simulink model "MSM_strain_wave_actuator"  (R2024b)
settings: Solver=ode23t  StartTime=0.0  StopTime=SIMULATION_TIME  FixedStep=MAX_TIME_STEP  MaxStep=MAX_TIME_STEP  RelTol=1e-3  AbsTol=1e-3  EnableMultiTasking=on
PreLoadFcn:
  | linear_mechanism = Simulink.Variant('motion_type == "linear"');
  | rotary_mechanism = Simulink.Variant('motion_type == "rotary"');
values from neighbouring files (symbols this model uses):
  action = round(out.position_data.Data(:,5))    [msm_tooth_training_run.m]
  contact_ratio = tooth_plates_cnt / (2 * (t_a / t_b + 1))    (= 2)    [MSM_mechanism_simulation_properties.m]
  contraction_initial = -msm_length * e_initial    (= -0.001)    [MSM_mechanism_simulation_properties.m]
  controller_type_vec = zeros(tooth_plates_cnt, 1)    [MSM_mechanism_simulation_properties.m]
  controller_velocity_setpoint = velocity_iter    [controller_mass_comparison_runs.m]
  disk_diameter = disk_teeth_count * tooth_pitch / pi    [MSM_mechanism_simulation_properties.m]    (also in msm_sim_runs_for_pid.m = evalin('base','disk_diameter'); save_sim_result.m = evalin('base','disk_diameter'))
  disk_height = 2.5e-4    (= 0.00025)    [MSM_mechanism_simulation_properties.m]    (also in get_tooth_properties.m)
  feedback_threshold = 1.025    [MSM_mechanism_simulation_properties.m]    (also in get_tooth_properties.m; msm_sim_runs_for_pid.m = evalin('base','feedback_threshold'))
  force_control_coeff = 1.0    (= 1)    [MSM_mechanism_simulation_properties.m]
  HALT_VELOCITY = 0.2    [MSM_mechanism_simulation_properties.m]    (also in get_tooth_properties.m)
  in_pair_angle_tooth_plates_pitch = 2*pi * (-2*tooth_pitch + in_pair_tooth_plates_pitch) / (pi*disk_diameter)    (= 0.412285714286)    [MSM_mechanism_simulation_properties.m]    (also in get_tooth_properties.m = 2*pi * (-2*tooth_pitch + in_pair_tooth_plates_pitch) / (pi*t)
  MAX_OVERLOAD_VELOCITY = 100    [MSM_mechanism_simulation_properties.m]    (also in get_tooth_properties.m)
  MAX_POSITION = rack_initial_position + max_teeth_passed * tooth_plates_cnt * angle_single_tooth_step    [MSM_mechanism_simulation_properties.m]    (also in get_tooth_properties.m)
  MAX_TIME_STEP = 5e-6    (= 5e-06)    [MSM_mechanism_simulation_properties.m]
  min_tooth_motion_range = -msm_length * allowed_elongation    (= -0.001)    [MSM_mechanism_simulation_properties.m]
  motion_type_number = NaN    [MSM_mechanism_simulation_properties.m]
  next_vec_fraction = -0.05    [MSM_mechanism_simulation_properties.m]    (also in msm_sim_runs_for_pid.m = evalin('base','next_vec_fraction'))
  obs_matrix = zeros(tooth_plates_cnt, obs_matrix_size)    [MSM_mechanism_simulation_properties.m]
  one_side_absolute_offset = one_side_elongation_capacity * msm_length    (= 0.0001)    [MSM_mechanism_simulation_properties.m]
  rack_coulumb_friction = 0.05    [MSM_mechanism_simulation_properties.m]
  rack_initial_position = rack_initial_position + 4*angle_single_tooth_step    (= 0.0554357142857)    [MSM_mechanism_simulation_properties.m]    (also in get_tooth_properties.m = rack_initial_position + 4*angle_single_tooth_step)
  rack_mass = 4e-3    (= 0.004)    [MSM_mechanism_simulation_properties.m]
  rotational_rack_coulumb_friction = rack_coulumb_friction * disk_diameter    (= 0.00175)    [MSM_mechanism_simulation_properties.m]
  SIMULATION_TIME = 0.06    [MSM_mechanism_simulation_properties.m]    (also in msm_actuation_time_sensetivity.m = 0.04; msm_sim_runs_for_pid.m = evalin('base','SIMULATION_TIME'); msm_simulation_run.m = 0.08; msm_tooth_training_run.m = 0.04)
  swing_block_tooth_plates_pitch = 2 * tooth_pitch * 22 + tooth_pitch / tooth_plates_cnt    (= 0.0172575)    [MSM_mechanism_simulation_properties.m]    (also in get_tooth_properties.m = 2 * tooth_pitch * 22 + tooth_pitch / tooth_plates_cnt)
  tooth_disk_mass = 5e-3    (= 0.005)    [MSM_mechanism_simulation_properties.m]
  tooth_pitch = tooth_pitch * tooth_size_modifier    (= 0.00039)    [MSM_mechanism_simulation_properties.m]    (also in get_tooth_properties.m = 0.00024661; msm_sim_runs_for_pid.m = evalin('base','tooth_pitch'); save_sim_result.m = evalin('base','tooth_pitch'))
  tooth_plates_cnt = 4    [MSM_mechanism_simulation_properties.m]    (also in MSM_simulation_data_processing.m = sim_data.tooth_plates_cnt; msm_actuation_time_sensetivity.m = plates_cnt_iter; msm_sim_runs_for_pid.m = evalin('base','tooth_plates_cnt'); msm_simulation_run.m = plates_cnt_iter)
  tooth_plates_pitch = tooth_pitch * 12 + tooth_pitch / tooth_plates_cnt    (= 0.0047775)    [MSM_mechanism_simulation_properties.m]    (also in get_tooth_properties.m = tooth_pitch * 12 + tooth_pitch / tooth_plates_cnt)
  useful_load = -2    [MSM_mechanism_simulation_properties.m]    (also in controller_mass_comparison_runs.m)
  useful_mass = 0.0001    [MSM_mechanism_simulation_properties.m]    (also in controller_mass_comparison_runs.m = 0.025)
  VALIDATION_START_TIME = 0.25*SIMULATION_TIME    (= 0.015)    [MSM_mechanism_simulation_properties.m]
  Z = griddata(x,y,z,X,Y)    [MSM_simulation_data_processing.m]
undefined symbols (not defined in the file or in its folder): controller_amplitude_setpoint, controller_desired_profile_type, controller_frequency_setpoint, controller_loop_type, enable_neighbours_obs, enable_vel_setpoint, external_control_value, has_external_controller, initial_spike_force, random_delay_probablity, random_switch_probability, sim_state_code, simulation_pause_time, X, Y
libraries: sm_lib x141, MSM_element x72, Flat_tooth_plate x36, Rotary_tooth_plate x36, Swing_mechanism x18, nesl_utility x16, simulink x10, fl_lib x9, rllib x7, spsMeanLib x2, slctrl_autotuning x2, slpidlib x1
(part 3 of 7)

== system MSM_strain_wave_actuator/controller/Closed//open loop simple feedback controller1 ==
  rack position : Inport
  position mapping : Inport  Port=2
  initial spike : Inport  Port=3
  VEC: Feedback threshold and next vec fraction : Inport  Port=4
  Velocity setpoint : Inport  Port=5
  Clock : Clock
  Constant : Constant  Value=tooth_pitch
  Constant1 : Constant  Value=1.5*MAX_TIME_STEP
  Data Type Conversion : DataTypeConversion  OutDataTypeStr=double  RndMeth=Round  SaturateOnIntegerOverflow=off
  Delay1 : Delay  DelayLength=1  InitialCondition=1
  Demux : Demux  Outputs=2
  Gain1 : Gain  Gain=force_control_coeff
  Loop type control : Constant  Value=controller_loop_type
  MATLAB Function : MATLAB Function  TreatAsAtomicUnit=on
  Relational Operator : RelationalOperator  Operator=~=  OutDataTypeStr=boolean  RndMeth=Simplest  InputSameDT=off
  Velocity to frequency : Product  Inputs=*/
  Control Input : Outport
  signal switch spike : Outport  Port=2
  wires:
  Constant1/1 -> MATLAB Function/4(initial_idle_time)
  Velocity to frequency/1 -> MATLAB Function/3(cycle_length)
  Loop type control/1 -> MATLAB Function/2(loop_type)
  MATLAB Function/1(output_vector) -> Gain1/1
  rack position/1 -> MATLAB Function/8(rack_position)
  MATLAB Function/2(cur_active_output) -> Delay1/1, Relational Operator/1
  Delay1/1 -> Relational Operator/2, MATLAB Function/10(currently_active)
  Clock/1 -> MATLAB Function/1(time)
  initial spike/1 -> MATLAB Function/9(ticks_cnt)
  position mapping/1 -> MATLAB Function/7(feedback)
  Gain1/1 -> Control Input/1
  Constant/1 -> Velocity to frequency/1
  Velocity setpoint/1 -> Velocity to frequency/2
  Demux/1 -> MATLAB Function/5(feedback_threshold)
  Demux/2 -> MATLAB Function/6(next_vec_fraction)
  VEC: Feedback threshold and next vec fraction/1 -> Demux/1
  Relational Operator/1 -> Data Type Conversion/1
  Data Type Conversion/1 -> signal switch spike/1

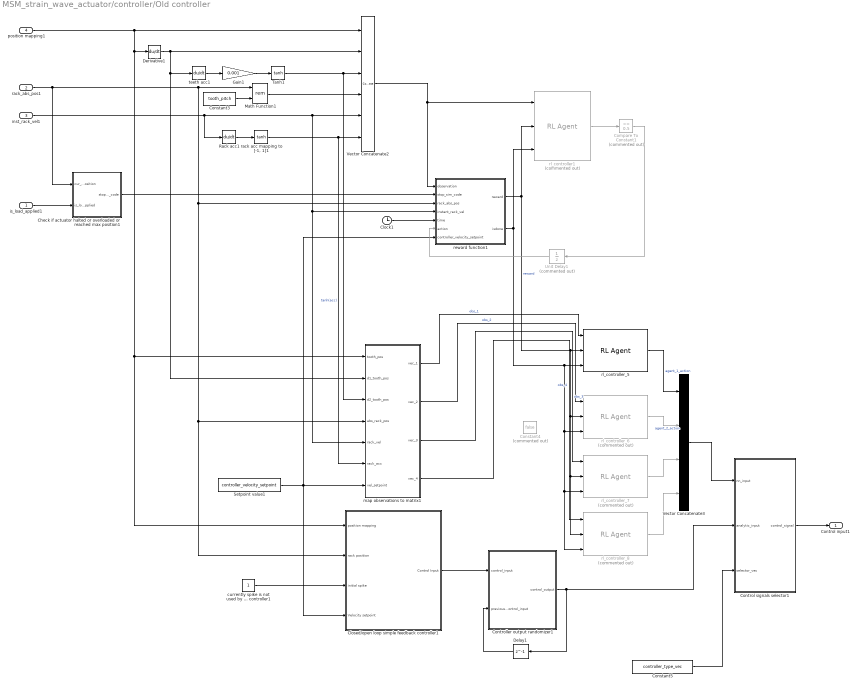
== system MSM_strain_wave_actuator/controller/Old controller ==
  is_load_applied1 : Inport
  rack_abs_pos1 : Inport  Port=2
  inst_rack_vel1 : Inport  Port=3
  position mapping1 : Inport  Port=4
  Check if actuator halted or overloaded or reached max position1 : Subsystem
  Clock1 : Clock
  Closed/open loop simple feedback controller1 : Subsystem
  Compare To Constant1 : simulink/Logic and Bit Operations/Compare To Constant  Commented=on  relop=>=  const=0.5  OutDataTypeStr=uint8
  Constant3 : Constant  Value=tooth_pitch
  Constant4 : Constant  Commented=on  Value=false
  Constant5 : Constant  Value=controller_type_vec
  Control signals selector1 : MATLAB Function  TreatAsAtomicUnit=on
  Controller output randomizer1 : MATLAB Function  TreatAsAtomicUnit=on
  Delay1 : Delay  DelayLength=1  InitialCondition=zeros(tooth_plates_cnt, 1)
  Derivative1 : Derivative
  Gain1 : Gain  Gain=0.001
  Math Function1 : Math  Operator=rem
  Rack acc1 : Derivative
  Setpoint value1 : Constant  Value=controller_velocity_setpoint
  Tanh1 : Trigonometry  Operator=tanh
  Unit Delay1 : UnitDelay  Commented=on  SampleTime=-1  HasFrameUpgradeWarning=on
  Vector Concatenate2 : Concatenate  NumInputs=6
  Vector Concatenate3 : Concatenate  NumInputs=4
  currently spike is not used by the controller1 : Constant
  map observations to matrix1 : MATLAB Function  TreatAsAtomicUnit=on
  "rack acc mapping to [-1, 1]1" : Trigonometry  Operator=tanh
  reward function1 : MATLAB Function  TreatAsAtomicUnit=on
  rl_controller1 : rllib/RL Agent  Commented=on  Agent=agent  ExternalActionAsInput=off  ProvideLastAction=off  ProvideCumRwd=off  TreatAsDirectFeedthrough=on  UseStrictObservationDataTypes=off
  rl_controller_5 : rllib/RL Agent  Agent=agent  ExternalActionAsInput=off  ProvideLastAction=off  ProvideCumRwd=off  TreatAsDirectFeedthrough=on  UseStrictObservationDataTypes=off
  rl_controller_6 : rllib/RL Agent  Commented=on  Agent=agent  ExternalActionAsInput=off  ProvideLastAction=off  ProvideCumRwd=off  TreatAsDirectFeedthrough=on  UseStrictObservationDataTypes=off
  rl_controller_7 : rllib/RL Agent  Commented=on  Agent=agent  ExternalActionAsInput=off  ProvideLastAction=off  ProvideCumRwd=off  TreatAsDirectFeedthrough=on  UseStrictObservationDataTypes=off
  rl_controller_8 : rllib/RL Agent  Commented=on  Agent=agent  ExternalActionAsInput=off  ProvideLastAction=off  ProvideCumRwd=off  TreatAsDirectFeedthrough=on  UseStrictObservationDataTypes=off
  teeth acc1 : Derivative
  Control input1 : Outport
  wires:
  inst_rack_vel1/1 -> Rack acc1/1, map observations to matrix1/5(rack_vel), reward function1/4(instant_rack_vel), Vector Concatenate2/5
  rl_controller1/1 -> Compare To Constant1/1
  Setpoint value1/1 -> reward function1/7(controller_velocity_setpoint), map observations to matrix1/7(vel_setpoint), Closed/open loop simple feedback controller1/4(Velocity setpoint)
  reward function1/1(reward) -> rl_controller1/2, rl_controller_7/2, rl_controller_8/2, rl_controller_6/2, rl_controller_5/2  "reward"
  Constant3/1 -> Math Function1/2
  Vector Concatenate2/1 -> reward function1/1(observation), rl_controller1/1
  reward function1/2(isdone) -> rl_controller1/3, rl_controller_8/3, rl_controller_7/3, rl_controller_6/3, rl_controller_5/3
  Controller output randomizer1/1(control_output) -> Control signals selector1/2(analytic_input), Delay1/1
  Compare To Constant1/1 -> Unit Delay1/1
  rack_abs_pos1/1 -> Check if actuator halted or overloaded or reached max position1/1(cur_rack_position), Closed/open loop simple feedback controller1/2(rack position), map observations to matrix1/4(abs_rack_pos), reward function1/3(rack_abs_pos), Math Function1/1
  Gain1/1 -> Tanh1/1
  Math Function1/1 -> Vector Concatenate2/4
  Unit Delay1/1 -> reward function1/6(action)
  currently spike is not used by the controller1/1 -> Closed/open loop simple feedback controller1/3(initial spike)
  map observations to matrix1/3(vec_3) -> rl_controller_7/1  "obs_3"
  position mapping1/1 -> Closed/open loop simple feedback controller1/1(position mapping), map observations to matrix1/1(tooth_pos), Derivative1/1, Vector Concatenate2/1
  map observations to matrix1/4(vec_4) -> rl_controller_8/1  "obs_4"
  is_load_applied1/1 -> Check if actuator halted or overloaded or reached max position1/2(is_load_applied)
  Vector Concatenate3/1 -> Control signals selector1/1(nn_input)
  Clock1/1 -> reward function1/5(time)
  "rack acc mapping to [-1, 1]1"/1 -> map observations to matrix1/6(rack_acc), Vector Concatenate2/6  "tanh(acc)"
  Tanh1/1 -> map observations to matrix1/3(d2_tooth_pos), Vector Concatenate2/3
  rl_controller_7/1 -> Vector Concatenate3/3
  rl_controller_8/1 -> Vector Concatenate3/4
  teeth acc1/1 -> Gain1/1
  map observations to matrix1/1(vec_1) -> rl_controller_5/1  "obs_1"
  rl_controller_6/1 -> Vector Concatenate3/2  "agent_2_action"
  Closed/open loop simple feedback controller1/1(Control Input) -> Controller output randomizer1/1(control_input)
  Control signals selector1/1(control_signal) -> Control input1/1
  map observations to matrix1/2(vec_2) -> rl_controller_6/1  "obs_2"
  Check if actuator halted or overloaded or reached max position1/1(stop_sim_code) -> reward function1/2(stop_sim_code)
  Constant5/1 -> Control signals selector1/3(selector_vec)
  Rack acc1/1 -> "rack acc mapping to [-1, 1]1"/1
  Delay1/1 -> Controller output randomizer1/2(previous_control_input)
  Derivative1/1 -> map observations to matrix1/2(d1_tooth_pos), teeth acc1/1, Vector Concatenate2/2
  rl_controller_5/1 -> Vector Concatenate3/1  "agent_1_action"

== system MSM_strain_wave_actuator/controller/Timing PID controller ==
  note: Feedback components:
      | rack pos
      | rack vel
      | rack acc [-1 1]
      | desired vel
  note: Notes on PID:
      | Average value as a feedback SIGNIFICANTLY reduces velocity oscilation. Plots comparison can be useful for the publication
      | Coeffs without average vel input: K=22, I=0.23
  feedback : Inport
  Constant : Constant  Value=0
  Constant1 : Constant
  Demux : Demux
  Derivative : Derivative
  Gain : Gain  Gain=35
  Gain1 : Gain  Gain=0.23
  Gain2 : Gain  Gain=0.01
  Integrator : Integrator
  Mux : Mux  Inputs=2
  PID controller : MATLAB Function  Commented=on  TreatAsAtomicUnit=on
  Sum : Sum  Inputs=|-+
  Sum1 : Sum  Inputs=++++
  control_vec : Outport
  wires:
  feedback/1 -> Demux/1
  Demux/4 -> Sum/2
  Sum/1 -> Derivative/1, Integrator/1, Gain/1
  Constant/1 -> Mux/2
  Mux/1 -> control_vec/1
  Integrator/1 -> Gain1/1
  Sum1/1 -> Mux/1
  Gain/1 -> Sum1/3
  Gain1/1 -> Sum1/2
  Constant1/1 -> Sum1/1
  Derivative/1 -> Gain2/1
  Gain2/1 -> Sum1/4
  Demux/2 -> Sum/1

== system MSM_strain_wave_actuator/controller/velocity via force ==
  note: Feedback components:
      | rack pos
      | rack vel
      | rack acc [-1 1]
      | desired vel
  note: Old Notes on PID for PWM (not in use anymore):
      | For L = 2,v=0.25 v=0.2, v=0.1
      | L = 1, v = 0.25
      | L = 0.5, v = 0.25 (somehow works, but extra tuning is needed)
      | P is relatively good up to value of 2
      | D is less than 1e-5 (not well tested)
      | I is around 17e+3
  feedback : Inport
  Closed-Loop PID Autotuner : slctrl_autotuning/Closed-Loop PID Autotuner  Commented=on  PIDType=PID  PIDForm=Parallel  TimeDomain=continuous-time  DiscreteTs=0.1  TuningTs=0.2  UseTuningTs=off  IntegratorFormula=Forward Euler  FilterFormula=Forward Euler  ContinuousTs=0.00005  Bandwidth=1000  UseExternalWC=off  TargetPM=60  UseExternalPM=off  UseExternalAchievedPM=off  ExperimentMode=Superposition  PlantType=Stable  PlantSign=Positive  AmpSine=0.01  UseExternalAmpSine=off  UseExternalFRD=off  UseExternalU0=off  UseCompanion=off  NotDeployTuningModule=off  UsePLCCoder=off  OutputMode=control action + perturbation  BlockDataType=double  UseConnectedPID=on  blockpath=[]  tunedP=0  tunedI=0  tunedD=0  tunedN=100  tunedPM=0  EstimationWindowSize=3  UseExternalTuningParams=off  SingleMultiRateVariant=SingleSamplingRate  NumEstimationPeriods=4  NumSettlingPeriods=2  NumOfPRBSPeriod=1  PRBSSignalOrder=12  ExperimentModeVariant=VariantSuperimposed  OutputChoice=VariantCandD  ConvergenceCalcVariant=ConvSuperpositionPRBSVariant
      settings: LibrarySourceBlock=slctrlblks/Autotuning/Closed-Loop PID Autotuner
  Constant : Constant  Commented=on
  Constant1 : Constant  Value=0.5
  Constant2 : Constant  Commented=on  Value=0
  Constant7 : Constant
  Demux : Demux
  Derivative : Derivative  Commented=on
  Discrete Derivative : simulink/Discrete/Discrete Derivative  gainval=1.0  ICPrevScaledInput=0.0  OutMin=[]  OutMax=[]  OutDataType=fixdt(1, 16)  OutScaling=2^-10  DoSatur=off
  Display : Display  Commented=on
  Display1 : Display  Commented=on
  Gain : Gain  Gain=6
  Gain1 : Gain  Gain=2e+4
  Gain2 : Gain  Gain=8e-5
  Gain3 : Gain  Gain=-1
  Gain4 : Gain  Gain=-1
  Integrator : Integrator
  Manual Switch : ManualSwitch  Commented=on
  Note: velocities are negative but output is positive that is why the input signs are flipped : Sum  Inputs=|+-
  Product : Product
  Sum1 : Sum  Inputs=++++
  does not owrk without this block It ensures the correct output sign : Signum  Commented=on
  PID force output : Outport
  wires:
  feedback/1 -> Demux/1
  Demux/4 -> Gain3/1
  Integrator/1 -> Gain1/1
  Gain/1 -> Sum1/3
  Constant1/1 -> Sum1/1
  Discrete Derivative/1 -> Gain2/1
  Gain4/1 -> Note: velocities are negative but output is positive that is why the input signs are flipped/2
  Gain3/1 -> does not owrk without this block It ensures the correct output sign/1, Note: velocities are negative but output is positive that is why the input signs are flipped/1
  Closed-Loop PID Autotuner/2 -> Display/1
  Closed-Loop PID Autotuner/3 -> Display1/1
  Constant/1 -> Manual Switch/2
  Constant2/1 -> Manual Switch/1
  Manual Switch/1 -> Closed-Loop PID Autotuner/3
  Gain1/1 -> Sum1/2  "error integral gain"
  Gain2/1 -> Sum1/4
  Demux/2 -> Gain4/1
  Sum1/1 -> Product/1
  Product/1 -> PID force output/1
  Constant7/1 -> Product/2
  Note: velocities are negative but output is positive that is why the input signs are flipped/1 -> Integrator/1, Discrete Derivative/1, Gain/1

== system MSM_strain_wave_actuator/controller/velocity via force1 ==
  note: Feedback components:
      | rack pos
      | rack vel
      | rack acc [-1 1]
      | desired vel
  note: Old Notes on PID for PWM (not in use anymore):
      | For L = 2,v=0.25 v=0.2, v=0.1
      | L = 1, v = 0.25
      | L = 0.5, v = 0.25 (somehow works, but extra tuning is needed)
      | P is relatively good up to value of 2
      | D is less than 1e-5 (not well tested)
      | I is around 17e+3
  feedback : Inport
  Closed-Loop PID Autotuner : slctrl_autotuning/Closed-Loop PID Autotuner  Commented=on  PIDType=PID  PIDForm=Parallel  TimeDomain=continuous-time  DiscreteTs=0.1  TuningTs=0.2  UseTuningTs=off  IntegratorFormula=Forward Euler  FilterFormula=Forward Euler  ContinuousTs=0.00005  Bandwidth=1000  UseExternalWC=off  TargetPM=60  UseExternalPM=off  UseExternalAchievedPM=off  ExperimentMode=Superposition  PlantType=Stable  PlantSign=Positive  AmpSine=0.01  UseExternalAmpSine=off  UseExternalFRD=off  UseExternalU0=off  UseCompanion=off  NotDeployTuningModule=off  UsePLCCoder=off  OutputMode=control action + perturbation  BlockDataType=double  UseConnectedPID=on  blockpath=[]  tunedP=0  tunedI=0  tunedD=0  tunedN=100  tunedPM=0  EstimationWindowSize=3  UseExternalTuningParams=off  SingleMultiRateVariant=SingleSamplingRate  NumEstimationPeriods=4  NumSettlingPeriods=2  NumOfPRBSPeriod=1  PRBSSignalOrder=12  ExperimentModeVariant=VariantSuperimposed  OutputChoice=VariantCandD  ConvergenceCalcVariant=ConvSuperpositionPRBSVariant
      settings: LibrarySourceBlock=slctrlblks/Autotuning/Closed-Loop PID Autotuner
  Constant : Constant  Commented=on
  Constant1 : Constant  Value=0.5
  Constant2 : Constant  Commented=on  Value=0
  Demux : Demux
  Derivative : Derivative  Commented=on
  Discrete Derivative : simulink/Discrete/Discrete Derivative  gainval=1.0  ICPrevScaledInput=0.0  OutMin=[]  OutMax=[]  OutDataType=fixdt(1, 16)  OutScaling=2^-10  DoSatur=off
  Display : Display  Commented=on
  Display1 : Display  Commented=on
  Gain : Gain  Gain=6
  Gain1 : Gain  Gain=2e+4
  Gain2 : Gain  Gain=8e-5
  Gain3 : Gain  Gain=-1
  Gain4 : Gain  Gain=-1
  Integrator : Integrator
  Manual Switch : ManualSwitch  Commented=on
  Note: velocities are negative but output is positive that is why the input signs are flipped : Sum  Inputs=|+-
  Sum1 : Sum  Inputs=++++
  PID force output : Outport
  wires:
  feedback/1 -> Demux/1
  Demux/4 -> Gain3/1
  Note: velocities are negative but output is positive that is why the input signs are flipped/1 -> Discrete Derivative/1, Integrator/1, Gain/1
  Integrator/1 -> Gain1/1
  Gain/1 -> Sum1/3
  Constant1/1 -> Sum1/1
  Discrete Derivative/1 -> Gain2/1
  Gain4/1 -> Note: velocities are negative but output is positive that is why the input signs are flipped/2, Closed-Loop PID Autotuner/2
  Gain3/1 -> Note: velocities are negative but output is positive that is why the input signs are flipped/1
  Closed-Loop PID Autotuner/2 -> Display/1
  Closed-Loop PID Autotuner/3 -> Display1/1
  Constant/1 -> Manual Switch/2
  Constant2/1 -> Manual Switch/1
  Manual Switch/1 -> Closed-Loop PID Autotuner/3
  Sum1/1 -> PID force output/1
  Gain1/1 -> Sum1/2  "error integral gain"
  Gain2/1 -> Sum1/4
  Demux/2 -> Gain4/1

== system MSM_strain_wave_actuator/MSM elements variant subsystem/Variable plate count Linear push push plates/Linear_swing_eight_tooth_plates ==
  Control input : Inport
  Demux : Demux  Outputs=8
  Mux : Mux  Inputs=8
  Rigid Transform1 : sm_lib/Frames and Transforms/Rigid Transform  RotationMethod=None  FollAlignAxisA=+X  BaseAlignAxisA=+Y  FollAlignAxisB=+Y  BaseAlignAxisB=+Z  RotationStandardAxis=+Z  RotationAngle=0.0  RotationAngleUnits=deg  RotationArbitraryAxis=[0 0 1]  RotationSequenceAxes=FollowerAxes  RotationSequence=XYX  RotationSequenceAngles=[0 0 0]  RotationSequenceAnglesUnits=deg  RotationMatrix=[1 0 0; 0 1 0; 0 0 1]  Quaternion=[1 0 0 0]  TranslationMethod=Cartesian  TranslationCartesianOffset=[swing_block_tooth_plates_pitch 0 0]  TranslationCartesianOffsetUnits=m  TranslationStandardAxis=+Z  TranslationStandardOffset=0  TranslationStandardOffsetUnits=m  TranslationROffset=0  TranslationROffsetUnits=m  TranslationThetaOffset=0  TranslationThetaOffsetUnits=deg  TranslationZOffset=0  TranslationZOffsetUnits=m
  Rigid Transform2 : sm_lib/Frames and Transforms/Rigid Transform  RotationMethod=None  FollAlignAxisA=+X  BaseAlignAxisA=+Y  FollAlignAxisB=+Y  BaseAlignAxisB=+Z  RotationStandardAxis=+Z  RotationAngle=0.0  RotationAngleUnits=deg  RotationArbitraryAxis=[0 0 1]  RotationSequenceAxes=FollowerAxes  RotationSequence=XYX  RotationSequenceAngles=[0 0 0]  RotationSequenceAnglesUnits=deg  RotationMatrix=[1 0 0; 0 1 0; 0 0 1]  Quaternion=[1 0 0 0]  TranslationMethod=Cartesian  TranslationCartesianOffset=[swing_block_tooth_plates_pitch 0 0]  TranslationCartesianOffsetUnits=m  TranslationStandardAxis=+Z  TranslationStandardOffset=0  TranslationStandardOffsetUnits=m  TranslationROffset=0  TranslationROffsetUnits=m  TranslationThetaOffset=0  TranslationThetaOffsetUnits=deg  TranslationZOffset=0  TranslationZOffsetUnits=m
  Rigid Transform3 : sm_lib/Frames and Transforms/Rigid Transform  RotationMethod=None  FollAlignAxisA=+X  BaseAlignAxisA=+Y  FollAlignAxisB=+Y  BaseAlignAxisB=+Z  RotationStandardAxis=+Z  RotationAngle=0.0  RotationAngleUnits=deg  RotationArbitraryAxis=[0 0 1]  RotationSequenceAxes=FollowerAxes  RotationSequence=XYX  RotationSequenceAngles=[0 0 0]  RotationSequenceAnglesUnits=deg  RotationMatrix=[1 0 0; 0 1 0; 0 0 1]  Quaternion=[1 0 0 0]  TranslationMethod=Cartesian  TranslationCartesianOffset=[swing_block_tooth_plates_pitch 0 0]  TranslationCartesianOffsetUnits=m  TranslationStandardAxis=+Z  TranslationStandardOffset=0  TranslationStandardOffsetUnits=m  TranslationROffset=0  TranslationROffsetUnits=m  TranslationThetaOffset=0  TranslationThetaOffsetUnits=deg  TranslationZOffset=0  TranslationZOffsetUnits=m
  Subsystem : Subsystem
  Subsystem1 : Subsystem
  Subsystem2 : Subsystem
  Subsystem3 : Subsystem
  Frame : PMIOPort  Side=Left
  Spatial force output : PMIOPort  Port=2  Side=Right
  Position Feedback : Outport
  Data output : Outport  Port=2
  wires:
  Control input/1 -> Demux/1
  Mux/1 -> Position Feedback/1
  Demux/1 -> Subsystem/1(Control input [0; 1])
  Subsystem/1(Tooth Position Unit 1) -> Mux/1
  Demux/2 -> Subsystem1/1(Control input [0; 1])
  Subsystem1/1(Tooth Position Unit 1) -> Mux/2
  Subsystem2/1(Tooth Position Unit 1) -> Mux/3
  Demux/3 -> Subsystem2/1(Control input [0; 1])
  Demux/4 -> Subsystem3/1(Control input [0; 1])
  Demux/5 -> Subsystem/2(Control input [0; 1]1)
  Demux/6 -> Subsystem1/2(Control input [0; 1]1)
  Demux/7 -> Subsystem2/2(Control input [0; 1]1)
  Demux/8 -> Subsystem3/2(Control input [0; 1]1)
  Subsystem3/1(Tooth Position Unit 1) -> Mux/4
  Subsystem/2("Tooth position COUNTERPHASE, mm") -> Mux/5
  Subsystem1/2("Tooth position COUNTERPHASE, mm") -> Mux/6
  Subsystem2/2("Tooth position COUNTERPHASE, mm") -> Mux/7
  Subsystem3/2("Tooth position COUNTERPHASE, mm") -> Mux/8
  connections:
  Subsystem2/RConn1 -- Subsystem3/RConn1 -- Subsystem1/RConn1 -- Spatial force output/RConn1 -- Subsystem/RConn1
  Rigid Transform1/LConn1 -- Subsystem/LConn1 -- Frame/RConn1
  Rigid Transform2/LConn1 -- Subsystem1/LConn1 -- Rigid Transform1/RConn1
  Rigid Transform2/RConn1 -- Rigid Transform3/LConn1 -- Subsystem2/LConn1
  Rigid Transform3/RConn1 -- Subsystem3/LConn1

== system MSM_strain_wave_actuator/MSM elements variant subsystem/Variable plate count Linear push push plates/Linear_swing_four_tooth_plates ==
  Control input : Inport
  Demux : Demux
  Mux : Mux
  Rigid Transform1 : sm_lib/Frames and Transforms/Rigid Transform  RotationMethod=None  FollAlignAxisA=+X  BaseAlignAxisA=+Y  FollAlignAxisB=+Y  BaseAlignAxisB=+Z  RotationStandardAxis=+Z  RotationAngle=0.0  RotationAngleUnits=deg  RotationArbitraryAxis=[0 0 1]  RotationSequenceAxes=FollowerAxes  RotationSequence=XYX  RotationSequenceAngles=[0 0 0]  RotationSequenceAnglesUnits=deg  RotationMatrix=[1 0 0; 0 1 0; 0 0 1]  Quaternion=[1 0 0 0]  TranslationMethod=Cartesian  TranslationCartesianOffset=[swing_block_tooth_plates_pitch 0 0]  TranslationCartesianOffsetUnits=m  TranslationStandardAxis=+Z  TranslationStandardOffset=0  TranslationStandardOffsetUnits=m  TranslationROffset=0  TranslationROffsetUnits=m  TranslationThetaOffset=0  TranslationThetaOffsetUnits=deg  TranslationZOffset=0  TranslationZOffsetUnits=m
  Subsystem : Subsystem
  Subsystem1 : Subsystem
  Frame : PMIOPort  Side=Left
  Spatial force output : PMIOPort  Port=2  Side=Right
  Position Feedback : Outport
  Data output : Outport  Port=2
  wires:
  Control input/1 -> Demux/1
  Mux/1 -> Position Feedback/1
  Demux/1 -> Subsystem/1(Control input [0; 1])
  Demux/3 -> Subsystem/2(Control input [0; 1]1)
  Subsystem/1(Tooth Position Unit 1) -> Mux/1
  Subsystem/2("Tooth position COUNTERPHASE, mm") -> Mux/3
  Demux/2 -> Subsystem1/1(Control input [0; 1])
  Demux/4 -> Subsystem1/2(Control input [0; 1]1)
  Subsystem1/1(Tooth Position Unit 1) -> Mux/2
  Subsystem1/2("Tooth position COUNTERPHASE, mm") -> Mux/4
  Subsystem/3(Data output) -> Data output/1
  connections:
  Spatial force output/RConn1 -- Subsystem/RConn1 -- Subsystem1/RConn1
  Rigid Transform1/LConn1 -- Frame/RConn1 -- Subsystem/LConn1
  Subsystem1/LConn1 -- Rigid Transform1/RConn1

== system MSM_strain_wave_actuator/MSM elements variant subsystem/Variable plate count Linear push push plates/Linear_swing_six_tooth_plates ==
  Control input : Inport
  Demux : Demux  Outputs=6
  Mux : Mux  Inputs=6
  Rigid Transform1 : sm_lib/Frames and Transforms/Rigid Transform  TranslationMethod=Cartesian  TranslationStandardOffset=0  TranslationStandardOffsetUnits=m  TranslationStandardAxis=+Z  TranslationCartesianOffset=[swing_block_tooth_plates_pitch 0 0]  TranslationCartesianOffsetUnits=m  TranslationROffset=0  TranslationROffsetUnits=m  TranslationZOffset=0  TranslationZOffsetUnits=m  TranslationThetaOffset=0  TranslationThetaOffsetUnits=deg  RotationMethod=None  RotationAngleUnits=deg  RotationStandardAxis=+Z  RotationAngle=0.0  RotationArbitraryAxis=[0 0 1]  FollAlignAxisA=+X  BaseAlignAxisA=+Y  FollAlignAxisB=+Y  BaseAlignAxisB=+Z  RotationSequenceAxes=FollowerAxes  RotationSequence=XYX  RotationSequenceAngles=[0 0 0]  RotationSequenceAnglesUnits=deg  RotationMatrix=[1 0 0; 0 1 0; 0 0 1]  Quaternion=[1 0 0 0]
  Rigid Transform2 : sm_lib/Frames and Transforms/Rigid Transform  TranslationMethod=Cartesian  TranslationStandardOffset=0  TranslationStandardOffsetUnits=m  TranslationStandardAxis=+Z  TranslationCartesianOffset=[swing_block_tooth_plates_pitch 0 0]  TranslationCartesianOffsetUnits=m  TranslationROffset=0  TranslationROffsetUnits=m  TranslationZOffset=0  TranslationZOffsetUnits=m  TranslationThetaOffset=0  TranslationThetaOffsetUnits=deg  RotationMethod=None  RotationAngleUnits=deg  RotationStandardAxis=+Z  RotationAngle=0.0  RotationArbitraryAxis=[0 0 1]  FollAlignAxisA=+X  BaseAlignAxisA=+Y  FollAlignAxisB=+Y  BaseAlignAxisB=+Z  RotationSequenceAxes=FollowerAxes  RotationSequence=XYX  RotationSequenceAngles=[0 0 0]  RotationSequenceAnglesUnits=deg  RotationMatrix=[1 0 0; 0 1 0; 0 0 1]  Quaternion=[1 0 0 0]
  Subsystem : Subsystem
  Subsystem1 : Subsystem
  Subsystem2 : Subsystem
  Frame : PMIOPort  Side=Left
  Spatial force output : PMIOPort  Port=2  Side=Right
  Position Feedback : Outport
  Data output : Outport  Port=2
  wires:
  Control input/1 -> Demux/1
  Mux/1 -> Position Feedback/1
  Demux/1 -> Subsystem/1(Control input [0; 1])
  Subsystem/1(Tooth Position Unit 1) -> Mux/1
  Demux/2 -> Subsystem1/1(Control input [0; 1])
  Subsystem1/1(Tooth Position Unit 1) -> Mux/2
  Subsystem/2("Tooth position COUNTERPHASE, mm") -> Mux/4
  Subsystem1/2("Tooth position COUNTERPHASE, mm") -> Mux/5
  Subsystem2/2("Tooth position COUNTERPHASE, mm") -> Mux/6
  Subsystem2/1(Tooth Position Unit 1) -> Mux/3
  Demux/4 -> Subsystem/2(Control input [0; 1]1)
  Demux/3 -> Subsystem2/1(Control input [0; 1])
  Demux/5 -> Subsystem1/2(Control input [0; 1]1)
  Demux/6 -> Subsystem2/2(Control input [0; 1]1)
  Subsystem/3(Data output) -> Data output/1
  connections:
  Spatial force output/RConn1 -- Subsystem/RConn1 -- Subsystem2/RConn1 -- Subsystem1/RConn1
  Rigid Transform1/LConn1 -- Subsystem/LConn1 -- Frame/RConn1
  Subsystem1/LConn1 -- Rigid Transform2/LConn1 -- Rigid Transform1/RConn1
  Rigid Transform2/RConn1 -- Subsystem2/LConn1

== system MSM_strain_wave_actuator/MSM elements variant subsystem/Variable plate count Rotary push push plates/Rotary push push 4 plates ==
  Control input : Inport
  Demux : Demux
  Mux1 : Mux
  Rigid Transform2 : sm_lib/Frames and Transforms/Rigid Transform  TranslationMethod=None  TranslationStandardOffset=0  TranslationStandardOffsetUnits=m  TranslationStandardAxis=+Z  TranslationCartesianOffset=[0 0 0]  TranslationCartesianOffsetUnits=m  TranslationROffset=0  TranslationROffsetUnits=m  TranslationZOffset=0  TranslationZOffsetUnits=m  TranslationThetaOffset=0  TranslationThetaOffsetUnits=deg  RotationMethod=StandardAxis  RotationAngleUnits=rad  RotationStandardAxis=+Z  RotationAngle=swing_block_angle_tooth_plates_pitch  RotationArbitraryAxis=[0 0 1]  FollAlignAxisA=+X  BaseAlignAxisA=+Y  FollAlignAxisB=+Y  BaseAlignAxisB=+Z  RotationSequenceAxes=FollowerAxes  RotationSequence=XYX  RotationSequenceAngles=[0 0 0]  RotationSequenceAnglesUnits=deg  RotationMatrix=[1 0 0; 0 1 0; 0 0 1]  Quaternion=[1 0 0 0]
  Subsystem : Subsystem
  Subsystem1 : Subsystem
  Spatial force output : PMIOPort  Side=Right
  Frame : PMIOPort  Port=2  Side=Left
  Position Feedback : Outport
  Data output : Outport  Port=2
  wires:
  Control input/1 -> Demux/1
  Mux1/1 -> Position Feedback/1
  Demux/1 -> Subsystem/1(Control input [0; 1])
  Subsystem/1("Tooth position, mm") -> Mux1/1
  Demux/2 -> Subsystem1/1(Control input [0; 1])
  Demux/3 -> Subsystem/2(Control input [0; 1]1)
  Demux/4 -> Subsystem1/2(Control input [0; 1]1)
  Subsystem1/1("Tooth position, mm") -> Mux1/2
  Subsystem/2("Tooth position, mm1") -> Mux1/3
  Subsystem1/2("Tooth position, mm1") -> Mux1/4
  Subsystem/3(Data output) -> Data output/1
  connections:
  Rigid Transform2/LConn1 -- Frame/RConn1 -- Subsystem/LConn1
  Spatial force output/RConn1 -- Subsystem1/RConn1 -- Subsystem/RConn1
  Rigid Transform2/RConn1 -- Subsystem1/LConn1

== system MSM_strain_wave_actuator/MSM elements variant subsystem/Variable plate count Rotary push push plates/Rotary push push 6 plates ==
  Control input : Inport
  Demux : Demux  Outputs=6
  Mux1 : Mux  Inputs=6
  Rigid Transform1 : sm_lib/Frames and Transforms/Rigid Transform  TranslationMethod=None  TranslationStandardOffset=0  TranslationStandardOffsetUnits=m  TranslationStandardAxis=+Z  TranslationCartesianOffset=[0 0 0]  TranslationCartesianOffsetUnits=m  TranslationROffset=0  TranslationROffsetUnits=m  TranslationZOffset=0  TranslationZOffsetUnits=m  TranslationThetaOffset=0  TranslationThetaOffsetUnits=deg  RotationMethod=StandardAxis  RotationAngleUnits=rad  RotationStandardAxis=+Z  RotationAngle=swing_block_angle_tooth_plates_pitch  RotationArbitraryAxis=[0 0 1]  FollAlignAxisA=+X  BaseAlignAxisA=+Y  FollAlignAxisB=+Y  BaseAlignAxisB=+Z  RotationSequenceAxes=FollowerAxes  RotationSequence=XYX  RotationSequenceAngles=[0 0 0]  RotationSequenceAnglesUnits=deg  RotationMatrix=[1 0 0; 0 1 0; 0 0 1]  Quaternion=[1 0 0 0]
  Rigid Transform2 : sm_lib/Frames and Transforms/Rigid Transform  TranslationMethod=None  TranslationStandardOffset=0  TranslationStandardOffsetUnits=m  TranslationStandardAxis=+Z  TranslationCartesianOffset=[0 0 0]  TranslationCartesianOffsetUnits=m  TranslationROffset=0  TranslationROffsetUnits=m  TranslationZOffset=0  TranslationZOffsetUnits=m  TranslationThetaOffset=0  TranslationThetaOffsetUnits=deg  RotationMethod=StandardAxis  RotationAngleUnits=rad  RotationStandardAxis=+Z  RotationAngle=swing_block_angle_tooth_plates_pitch  RotationArbitraryAxis=[0 0 1]  FollAlignAxisA=+X  BaseAlignAxisA=+Y  FollAlignAxisB=+Y  BaseAlignAxisB=+Z  RotationSequenceAxes=FollowerAxes  RotationSequence=XYX  RotationSequenceAngles=[0 0 0]  RotationSequenceAnglesUnits=deg  RotationMatrix=[1 0 0; 0 1 0; 0 0 1]  Quaternion=[1 0 0 0]
  Subsystem : Subsystem
  Subsystem1 : Subsystem
  Subsystem2 : Subsystem
  Spatial force output : PMIOPort  Side=Right
  Frame : PMIOPort  Port=2  Side=Left
  Position Feedback : Outport
  Data output : Outport  Port=2
  wires:
  Control input/1 -> Demux/1
  Mux1/1 -> Position Feedback/1
  Demux/1 -> Subsystem/1(Control input [0; 1])
  Subsystem/1("Tooth position, mm") -> Mux1/1
  Demux/2 -> Subsystem1/1(Control input [0; 1])
  Demux/3 -> Subsystem2/1(Control input [0; 1])
  Demux/4 -> Subsystem/2(Control input [0; 1]1)
  Demux/5 -> Subsystem1/2(Control input [0; 1]1)
  Demux/6 -> Subsystem2/2(Control input [0; 1]1)
  Subsystem1/1("Tooth position, mm") -> Mux1/2
  Subsystem2/1("Tooth position, mm") -> Mux1/3
  Subsystem/2("Tooth position, mm1") -> Mux1/4
  Subsystem1/2("Tooth position, mm1") -> Mux1/5
  Subsystem2/2("Tooth position, mm1") -> Mux1/6
  Subsystem/3(Data output) -> Data output/1
  connections:
  Rigid Transform2/LConn1 -- Frame/RConn1 -- Subsystem/LConn1
  Spatial force output/RConn1 -- Subsystem2/RConn1 -- Subsystem1/RConn1 -- Subsystem/RConn1
  Rigid Transform2/RConn1 -- Rigid Transform1/LConn1 -- Subsystem1/LConn1
  Rigid Transform1/RConn1 -- Subsystem2/LConn1

== system MSM_strain_wave_actuator/MSM elements variant subsystem/Variable plate count Rotary push push plates/Rotary push push 8 plates ==
  Control input : Inport
  Demux : Demux  Outputs=8
  Mux1 : Mux  Inputs=8
  Rigid Transform1 : sm_lib/Frames and Transforms/Rigid Transform  TranslationMethod=None  TranslationStandardOffset=0  TranslationStandardOffsetUnits=m  TranslationStandardAxis=+Z  TranslationCartesianOffset=[0 0 0]  TranslationCartesianOffsetUnits=m  TranslationROffset=0  TranslationROffsetUnits=m  TranslationZOffset=0  TranslationZOffsetUnits=m  TranslationThetaOffset=0  TranslationThetaOffsetUnits=deg  RotationMethod=StandardAxis  RotationAngleUnits=rad  RotationStandardAxis=+Z  RotationAngle=swing_block_angle_tooth_plates_pitch  RotationArbitraryAxis=[0 0 1]  FollAlignAxisA=+X  BaseAlignAxisA=+Y  FollAlignAxisB=+Y  BaseAlignAxisB=+Z  RotationSequenceAxes=FollowerAxes  RotationSequence=XYX  RotationSequenceAngles=[0 0 0]  RotationSequenceAnglesUnits=deg  RotationMatrix=[1 0 0; 0 1 0; 0 0 1]  Quaternion=[1 0 0 0]
  Rigid Transform2 : sm_lib/Frames and Transforms/Rigid Transform  TranslationMethod=None  TranslationStandardOffset=0  TranslationStandardOffsetUnits=m  TranslationStandardAxis=+Z  TranslationCartesianOffset=[0 0 0]  TranslationCartesianOffsetUnits=m  TranslationROffset=0  TranslationROffsetUnits=m  TranslationZOffset=0  TranslationZOffsetUnits=m  TranslationThetaOffset=0  TranslationThetaOffsetUnits=deg  RotationMethod=StandardAxis  RotationAngleUnits=rad  RotationStandardAxis=+Z  RotationAngle=swing_block_angle_tooth_plates_pitch  RotationArbitraryAxis=[0 0 1]  FollAlignAxisA=+X  BaseAlignAxisA=+Y  FollAlignAxisB=+Y  BaseAlignAxisB=+Z  RotationSequenceAxes=FollowerAxes  RotationSequence=XYX  RotationSequenceAngles=[0 0 0]  RotationSequenceAnglesUnits=deg  RotationMatrix=[1 0 0; 0 1 0; 0 0 1]  Quaternion=[1 0 0 0]
  Rigid Transform3 : sm_lib/Frames and Transforms/Rigid Transform  TranslationMethod=None  TranslationStandardOffset=0  TranslationStandardOffsetUnits=m  TranslationStandardAxis=+Z  TranslationCartesianOffset=[0 0 0]  TranslationCartesianOffsetUnits=m  TranslationROffset=0  TranslationROffsetUnits=m  TranslationZOffset=0  TranslationZOffsetUnits=m  TranslationThetaOffset=0  TranslationThetaOffsetUnits=deg  RotationMethod=StandardAxis  RotationAngleUnits=rad  RotationStandardAxis=+Z  RotationAngle=swing_block_angle_tooth_plates_pitch  RotationArbitraryAxis=[0 0 1]  FollAlignAxisA=+X  BaseAlignAxisA=+Y  FollAlignAxisB=+Y  BaseAlignAxisB=+Z  RotationSequenceAxes=FollowerAxes  RotationSequence=XYX  RotationSequenceAngles=[0 0 0]  RotationSequenceAnglesUnits=deg  RotationMatrix=[1 0 0; 0 1 0; 0 0 1]  Quaternion=[1 0 0 0]
  Subsystem : Subsystem
  Subsystem1 : Subsystem
  Subsystem2 : Subsystem
  Subsystem3 : Subsystem
  Spatial force output : PMIOPort  Side=Right
  Frame : PMIOPort  Port=2  Side=Left
  Position Feedback : Outport
  Data output : Outport  Port=2
  wires:
  Control input/1 -> Demux/1
  Mux1/1 -> Position Feedback/1
  Demux/1 -> Subsystem/1(Control input [0; 1])
  Subsystem/1("Tooth position, mm") -> Mux1/1
  Demux/2 -> Subsystem1/1(Control input [0; 1])
  Subsystem1/1("Tooth position, mm") -> Mux1/2
  Demux/3 -> Subsystem2/1(Control input [0; 1])
  Demux/4 -> Subsystem3/1(Control input [0; 1])
  Demux/5 -> Subsystem/2(Control input [0; 1]1)
  Demux/6 -> Subsystem1/2(Control input [0; 1]1)
  Demux/7 -> Subsystem2/2(Control input [0; 1]1)
  Demux/8 -> Subsystem3/2(Control input [0; 1]1)
  Subsystem2/1("Tooth position, mm") -> Mux1/3
  Subsystem3/1("Tooth position, mm") -> Mux1/4
  Subsystem/2("Tooth position, mm1") -> Mux1/5
  Subsystem1/2("Tooth position, mm1") -> Mux1/6
  Subsystem2/2("Tooth position, mm1") -> Mux1/7
  Subsystem3/2("Tooth position, mm1") -> Mux1/8
  Subsystem/3(Data output) -> Data output/1
  connections:
  Rigid Transform2/LConn1 -- Frame/RConn1 -- Subsystem/LConn1
  Spatial force output/RConn1 -- Subsystem3/RConn1 -- Subsystem2/RConn1 -- Subsystem1/RConn1 -- Subsystem/RConn1
  Rigid Transform2/RConn1 -- Subsystem1/LConn1 -- Rigid Transform1/LConn1
  Rigid Transform1/RConn1 -- Rigid Transform3/LConn1 -- Subsystem2/LConn1
  Rigid Transform3/RConn1 -- Subsystem3/LConn1

== system MSM_strain_wave_actuator/MSM elements variant subsystem/Variable plate count Rotary push spring plates/Rotary push spring 4 plates ==
  Control input : Inport
  Demux : Demux
  MSM and tooth plate{1..4} (4 alike) : MSM_element/MSM and tooth plate  PositionTargetValue=contraction_initial
  MSM plate translation{,1..3} (4 alike) : sm_lib/Frames and Transforms/Rigid Transform  TranslationMethod=StandardAxis  TranslationStandardOffset=disk_diameter / 2  TranslationStandardOffsetUnits=m  TranslationStandardAxis=+Y  TranslationCartesianOffset=[0 0 0]  TranslationCartesianOffsetUnits=m  TranslationROffset=0  TranslationROffsetUnits=m  TranslationZOffset=0  TranslationZOffsetUnits=m  TranslationThetaOffset=0  TranslationThetaOffsetUnits=deg  RotationMethod=StandardAxis  RotationAngleUnits=deg  RotationStandardAxis=-X  RotationAngle=90  RotationArbitraryAxis=[0 0 1]  FollAlignAxisA=+X  BaseAlignAxisA=+Y  FollAlignAxisB=+Y  BaseAlignAxisB=+Z  RotationSequenceAxes=FollowerAxes  RotationSequence=XYX  RotationSequenceAngles=[0 0 0]  RotationSequenceAnglesUnits=deg  RotationMatrix=[1 0 0; 0 1 0; 0 0 1]  Quaternion=[1 0 0 0]
  Mux1 : Mux
  Mux2 : Mux  Inputs=7
  Rigid Transform : sm_lib/Frames and Transforms/Rigid Transform  TranslationMethod=None  TranslationStandardOffset=0  TranslationStandardOffsetUnits=m  TranslationStandardAxis=+Z  TranslationCartesianOffset=[0 0 0]  TranslationCartesianOffsetUnits=m  TranslationROffset=0  TranslationROffsetUnits=m  TranslationZOffset=0  TranslationZOffsetUnits=m  TranslationThetaOffset=0  TranslationThetaOffsetUnits=deg  RotationMethod=StandardAxis  RotationAngleUnits=rad  RotationStandardAxis=+Z  RotationAngle=angle_tooth_plates_pitch  RotationArbitraryAxis=[0 0 1]  FollAlignAxisA=+X  BaseAlignAxisA=+Y  FollAlignAxisB=+Y  BaseAlignAxisB=+Z  RotationSequenceAxes=FollowerAxes  RotationSequence=XYX  RotationSequenceAngles=[0 0 0]  RotationSequenceAnglesUnits=deg  RotationMatrix=[1 0 0; 0 1 0; 0 0 1]  Quaternion=[1 0 0 0]
  Rigid Transform1 : sm_lib/Frames and Transforms/Rigid Transform  TranslationMethod=None  TranslationStandardOffset=0  TranslationStandardOffsetUnits=m  TranslationStandardAxis=+Z  TranslationCartesianOffset=[0 0 0]  TranslationCartesianOffsetUnits=m  TranslationROffset=0  TranslationROffsetUnits=m  TranslationZOffset=0  TranslationZOffsetUnits=m  TranslationThetaOffset=0  TranslationThetaOffsetUnits=deg  RotationMethod=StandardAxis  RotationAngleUnits=rad  RotationStandardAxis=+Z  RotationAngle=angle_tooth_plates_pitch  RotationArbitraryAxis=[0 0 1]  FollAlignAxisA=+X  BaseAlignAxisA=+Y  FollAlignAxisB=+Y  BaseAlignAxisB=+Z  RotationSequenceAxes=FollowerAxes  RotationSequence=XYX  RotationSequenceAngles=[0 0 0]  RotationSequenceAnglesUnits=deg  RotationMatrix=[1 0 0; 0 1 0; 0 0 1]  Quaternion=[1 0 0 0]
  Rigid Transform2 : sm_lib/Frames and Transforms/Rigid Transform  TranslationMethod=None  TranslationStandardOffset=0  TranslationStandardOffsetUnits=m  TranslationStandardAxis=+Z  TranslationCartesianOffset=[0 0 0]  TranslationCartesianOffsetUnits=m  TranslationROffset=0  TranslationROffsetUnits=m  TranslationZOffset=0  TranslationZOffsetUnits=m  TranslationThetaOffset=0  TranslationThetaOffsetUnits=deg  RotationMethod=StandardAxis  RotationAngleUnits=rad  RotationStandardAxis=+Z  RotationAngle=angle_tooth_plates_pitch  RotationArbitraryAxis=[0 0 1]  FollAlignAxisA=+X  BaseAlignAxisA=+Y  FollAlignAxisB=+Y  BaseAlignAxisB=+Z  RotationSequenceAxes=FollowerAxes  RotationSequence=XYX  RotationSequenceAngles=[0 0 0]  RotationSequenceAnglesUnits=deg  RotationMatrix=[1 0 0; 0 1 0; 0 0 1]  Quaternion=[1 0 0 0]
  Rotary_tooth_plate{,1..3} (4 alike) : Rotary_tooth_plate/Rotary_tooth_plate  SystemSampleTime=-1  VariantActivationTime=update diagram  AllowFlexibleInterface=on  Latency=0  AutoFrameSizeCalculation=off
  Spatial force output : PMIOPort  Side=Right
  Frame : PMIOPort  Port=2  Side=Left
  Position Feedback : Outport
  Data output : Outport  Port=2
  wires:
  Demux/4 -> MSM and tooth plate4/1
  MSM and tooth plate2/1 -> Mux1/2
  Control input/1 -> Demux/1
  Mux1/1 -> Position Feedback/1
  Demux/3 -> MSM and tooth plate3/1
  MSM and tooth plate4/1 -> Mux1/4
  Demux/1 -> MSM and tooth plate1/1
  Demux/2 -> MSM and tooth plate2/1
  MSM and tooth plate3/1 -> Mux1/3
  MSM and tooth plate1/1 -> Mux2/1, Mux1/1
  Mux2/1 -> Data output/1
  MSM and tooth plate1/2 -> Mux2/2
  MSM and tooth plate1/3 -> Mux2/3
  MSM and tooth plate1/4 -> Mux2/4
  MSM and tooth plate1/5 -> Mux2/5
  MSM and tooth plate1/7 -> Mux2/6
  MSM and tooth plate1/8 -> Mux2/7
  connections:
  MSM plate translation/RConn1 -- Rotary_tooth_plate/LConn2 -- MSM and tooth plate4/LConn1
  MSM plate translation3/LConn1 -- Rigid Transform/LConn1 -- Rigid Transform2/RConn1
  MSM plate translation1/LConn1 -- Frame/RConn1 -- Rigid Transform1/LConn1
  Rotary_tooth_plate1/RConn1 -- Spatial force output/RConn1 -- Rotary_tooth_plate2/RConn1 -- Rotary_tooth_plate/RConn1 -- Rotary_tooth_plate3/RConn1
  MSM and tooth plate4/RConn1 -- Rotary_tooth_plate/LConn1
  MSM and tooth plate1/RConn1 -- Rotary_tooth_plate1/LConn1
  Rotary_tooth_plate1/LConn2 -- MSM plate translation1/RConn1 -- MSM and tooth plate1/LConn1
  MSM plate translation2/LConn1 -- Rigid Transform2/LConn1 -- Rigid Transform1/RConn1
  MSM and tooth plate2/RConn1 -- Rotary_tooth_plate2/LConn1
  MSM plate translation/LConn1 -- Rigid Transform/RConn1
  MSM and tooth plate3/RConn1 -- Rotary_tooth_plate3/LConn1
  MSM plate translation3/RConn1 -- Rotary_tooth_plate3/LConn2 -- MSM and tooth plate3/LConn1
  MSM plate translation2/RConn1 -- Rotary_tooth_plate2/LConn2 -- MSM and tooth plate2/LConn1

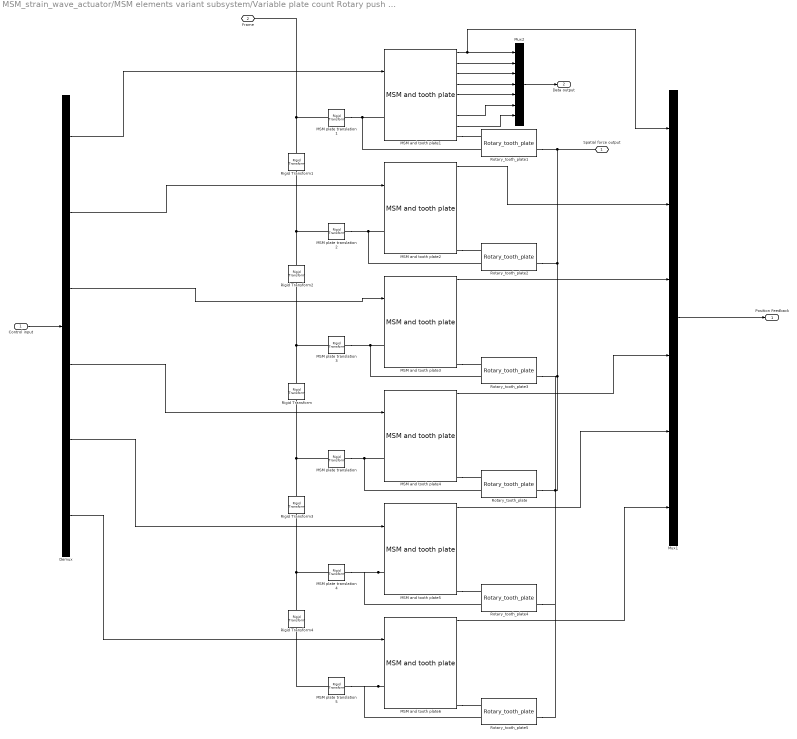
== system MSM_strain_wave_actuator/MSM elements variant subsystem/Variable plate count Rotary push spring plates/Rotary push spring 6 plates ==
  Control input : Inport
  Demux : Demux  Outputs=6
  MSM and tooth plate{1..6} (6 alike) : MSM_element/MSM and tooth plate  PositionTargetValue=contraction_initial
  MSM plate translation{,1..5} (6 alike) : sm_lib/Frames and Transforms/Rigid Transform  TranslationMethod=StandardAxis  TranslationStandardOffset=disk_diameter / 2  TranslationStandardOffsetUnits=m  TranslationStandardAxis=+Y  TranslationCartesianOffset=[0 0 0]  TranslationCartesianOffsetUnits=m  TranslationROffset=0  TranslationROffsetUnits=m  TranslationZOffset=0  TranslationZOffsetUnits=m  TranslationThetaOffset=0  TranslationThetaOffsetUnits=deg  RotationMethod=StandardAxis  RotationAngleUnits=deg  RotationStandardAxis=-X  RotationAngle=90  RotationArbitraryAxis=[0 0 1]  FollAlignAxisA=+X  BaseAlignAxisA=+Y  FollAlignAxisB=+Y  BaseAlignAxisB=+Z  RotationSequenceAxes=FollowerAxes  RotationSequence=XYX  RotationSequenceAngles=[0 0 0]  RotationSequenceAnglesUnits=deg  RotationMatrix=[1 0 0; 0 1 0; 0 0 1]  Quaternion=[1 0 0 0]
  Mux1 : Mux  Inputs=6
  Mux2 : Mux  Inputs=7
  Rigid Transform{,1..4} (5 alike) : sm_lib/Frames and Transforms/Rigid Transform  TranslationMethod=None  TranslationStandardOffset=0  TranslationStandardOffsetUnits=m  TranslationStandardAxis=+Z  TranslationCartesianOffset=[0 0 0]  TranslationCartesianOffsetUnits=m  TranslationROffset=0  TranslationROffsetUnits=m  TranslationZOffset=0  TranslationZOffsetUnits=m  TranslationThetaOffset=0  TranslationThetaOffsetUnits=deg  RotationMethod=StandardAxis  RotationAngleUnits=rad  RotationStandardAxis=+Z  RotationAngle=angle_tooth_plates_pitch  RotationArbitraryAxis=[0 0 1]  FollAlignAxisA=+X  BaseAlignAxisA=+Y  FollAlignAxisB=+Y  BaseAlignAxisB=+Z  RotationSequenceAxes=FollowerAxes  RotationSequence=XYX  RotationSequenceAngles=[0 0 0]  RotationSequenceAnglesUnits=deg  RotationMatrix=[1 0 0; 0 1 0; 0 0 1]  Quaternion=[1 0 0 0]
  Rotary_tooth_plate{,1..5} (6 alike) : Rotary_tooth_plate/Rotary_tooth_plate  SystemSampleTime=-1  VariantActivationTime=update diagram  AllowFlexibleInterface=on  Latency=0  AutoFrameSizeCalculation=off
  Spatial force output : PMIOPort  Side=Right
  Frame : PMIOPort  Port=2  Side=Left
  Position Feedback : Outport
  Data output : Outport  Port=2
  wires:
  Demux/4 -> MSM and tooth plate4/1
  MSM and tooth plate2/1 -> Mux1/2
  Control input/1 -> Demux/1
  Mux1/1 -> Position Feedback/1
  Demux/3 -> MSM and tooth plate3/1
  MSM and tooth plate4/1 -> Mux1/4
  Demux/1 -> MSM and tooth plate1/1
  Demux/2 -> MSM and tooth plate2/1
  MSM and tooth plate3/1 -> Mux1/3
  MSM and tooth plate1/1 -> Mux2/1, Mux1/1
  Demux/5 -> MSM and tooth plate5/1
  Demux/6 -> MSM and tooth plate6/1
  MSM and tooth plate5/1 -> Mux1/5
  MSM and tooth plate6/1 -> Mux1/6
  Mux2/1 -> Data output/1
  MSM and tooth plate1/2 -> Mux2/2
  MSM and tooth plate1/3 -> Mux2/3
  MSM and tooth plate1/4 -> Mux2/4
  MSM and tooth plate1/5 -> Mux2/5
  MSM and tooth plate1/7 -> Mux2/6
  MSM and tooth plate1/8 -> Mux2/7
  connections:
  MSM plate translation/RConn1 -- Rotary_tooth_plate/LConn2 -- MSM and tooth plate4/LConn1
  MSM plate translation3/LConn1 -- Rigid Transform/LConn1 -- Rigid Transform2/RConn1
  MSM plate translation1/LConn1 -- Frame/RConn1 -- Rigid Transform1/LConn1
  Rotary_tooth_plate1/RConn1 -- Spatial force output/RConn1 -- Rotary_tooth_plate2/RConn1 -- Rotary_tooth_plate5/RConn1 -- Rotary_tooth_plate4/RConn1 -- Rotary_tooth_plate/RConn1 -- Rotary_tooth_plate3/RConn1
  MSM and tooth plate4/RConn1 -- Rotary_tooth_plate/LConn1
  MSM and tooth plate1/RConn1 -- Rotary_tooth_plate1/LConn1
  Rotary_tooth_plate1/LConn2 -- MSM plate translation1/RConn1 -- MSM and tooth plate1/LConn1
  MSM plate translation2/LConn1 -- Rigid Transform2/LConn1 -- Rigid Transform1/RConn1
  MSM and tooth plate2/RConn1 -- Rotary_tooth_plate2/LConn1
  MSM plate translation/LConn1 -- Rigid Transform3/LConn1 -- Rigid Transform/RConn1
  MSM and tooth plate3/RConn1 -- Rotary_tooth_plate3/LConn1
  MSM plate translation3/RConn1 -- Rotary_tooth_plate3/LConn2 -- MSM and tooth plate3/LConn1
  MSM plate translation2/RConn1 -- Rotary_tooth_plate2/LConn2 -- MSM and tooth plate2/LConn1
  MSM and tooth plate5/LConn1 -- MSM plate translation4/RConn1 -- Rotary_tooth_plate4/LConn2
  MSM plate translation4/LConn1 -- Rigid Transform3/RConn1 -- Rigid Transform4/LConn1
  MSM and tooth plate5/RConn1 -- Rotary_tooth_plate4/LConn1
  MSM and tooth plate6/LConn1 -- MSM plate translation5/RConn1 -- Rotary_tooth_plate5/LConn2
  MSM plate translation5/LConn1 -- Rigid Transform4/RConn1
  MSM and tooth plate6/RConn1 -- Rotary_tooth_plate5/LConn1
